simulink model "simula_epsac"  (R2018a)
settings: Solver=VariableStepAuto  StartTime=0.0  StopTime=Tsim  RelTol=1e-3
values from neighbouring files (symbols this model uses):
  GPC = gpc_tf2ss_U(Pz,[],delta,n,nu)    [espac_generic.m]
  Ql = 0.8*eye(nu)    [espac_generic.m]
  Ts = 1    [espac_generic.m]
  Tsim = 35    [espac_generic.m]
undefined symbols (not defined in the file or in its folder): Qd
libraries: simulink x1, cstblocks x1
settings Model: Creator=marcus  LastModifiedBy=marcus

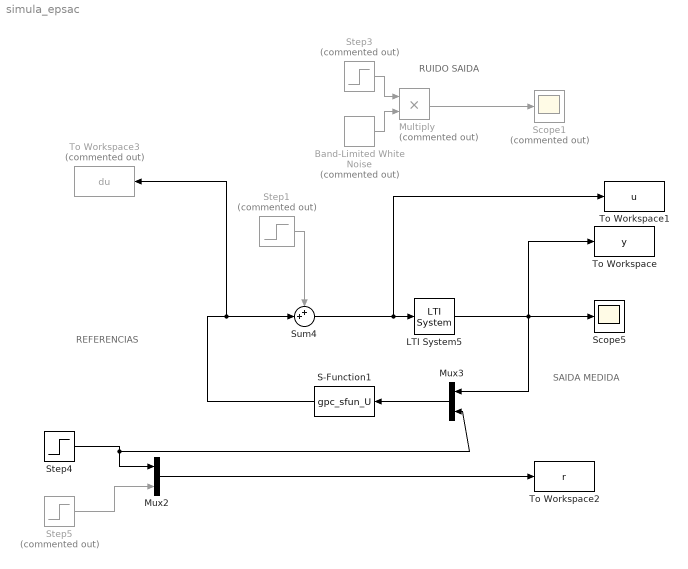
== system simula_epsac ==
  note: SAIDA MEDIDA
  note: REFERENCIAS
  note: RUIDO SAIDA
  Band-Limited White Noise : simulink/Sources/Band-Limited White Noise  Commented=on  Cov=Ts/5000  Ts=Ts/10  seed=[23341]
  LTI System5 : cstblocks/LTI System  sys=P  IC=[]
  Multiply : Product  Commented=on
  Mux2 : Mux  Inputs=2
  Mux3 : Mux  Inputs=2
  S-Function1 : S-Function  FunctionName=gpc_sfun_U  Parameters=GPC,Ql,Qd  SFunctionDeploymentMode=off  EnableBusSupport=off
  Scope1 : Scope  Commented=on
  Scope5 : Scope
  Step1 : Step  Commented=on  Time=Tsim/2  SampleTime=0
  Step3 : Step  Commented=on  Time=4*Tsim/5  SampleTime=0
  Step4 : Step  Time=0  SampleTime=Ts
  Step5 : Step  Commented=on  Time=0  After=0.2  SampleTime=Ts
  Sum4 : Sum  Inputs=++|
  To Workspace : ToWorkspace  VariableName=y  SaveFormat=Timeseries  SampleTime=Ts
  To Workspace1 : ToWorkspace  VariableName=u  SaveFormat=Timeseries  SampleTime=Ts
  To Workspace2 : ToWorkspace  VariableName=r  SaveFormat=Timeseries  SampleTime=-1
  To Workspace3 : ToWorkspace  Commented=on  VariableName=du  SaveFormat=Timeseries  SampleTime=Ts
  wires:
  Mux2/1 -> To Workspace2/1
  Mux3/1 -> S-Function1/1
  Sum4/1 -> To Workspace1/1, LTI System5/1
  S-Function1/1 -> Sum4/2, To Workspace3/1
  Step1/1 -> Sum4/1
  Step3/1 -> Multiply/1
  Band-Limited White Noise/1 -> Multiply/2
  LTI System5/1 -> To Workspace/1, Mux3/1, Scope5/1
  Step4/1 -> Mux3/2, Mux2/1
  Multiply/1 -> Scope1/1
  Step5/1 -> Mux2/2
